simulink model "test_staticRelief"  (R2013a)
settings: Solver=ode15s  StartTime=0.0  StopTime=3  RelTol=1e-5
libraries: fl_lib x5, nesl_utility x3, simulink x2, usask_hyd_lib x1
settings Model: Creator=tkw954  LastModifiedBy=tkw954

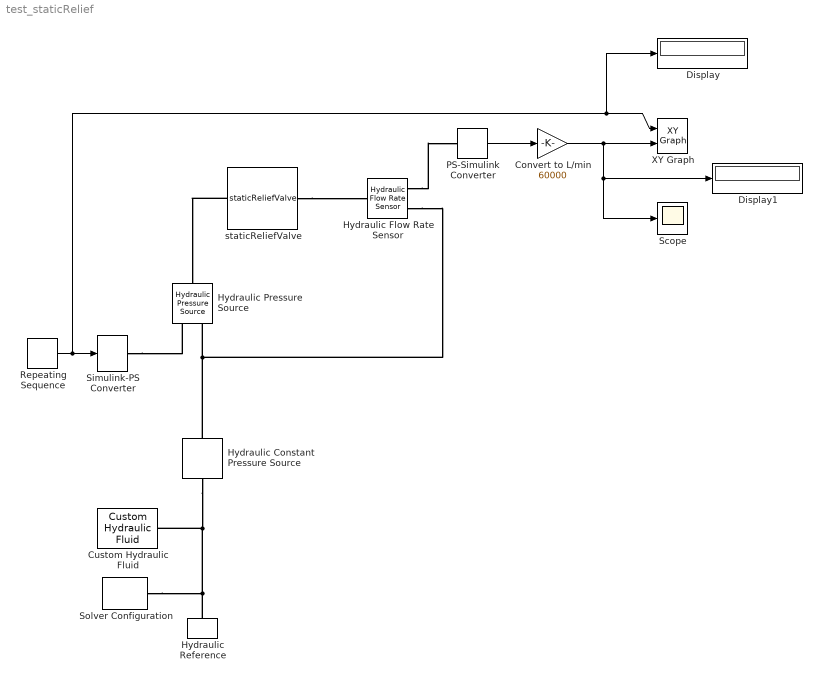
== system test_staticRelief ==
  Convert to L/min : Gain  Gain=60000
  Custom Hydraulic Fluid : fl_lib/Hydraulic/Hydraulic Utilities/Custom Hydraulic Fluid  density=850 kg/m^3  viscosity_kin=18e-6 m^2/s  bulk=0.8e9 Pa  alpha=0.005  LocalVarLogging=[]
  Display : Display
  Display1 : Display
  Hydraulic Constant Pressure Source : fl_lib/Hydraulic/Hydraulic Sources/Hydraulic Constant Pressure Source  commanded_pressure=10e6 Pa  pressure_Log=off  flow_rate_Log=off  power_Log=off  LocalVarNames=|pressure|flow_rate|power  LocalVarDescs=|Pressure differential|Flow rate|Power generated by the source  LocalVarLogging=[0 0 0]
  Hydraulic Flow Rate Sensor : fl_lib/Hydraulic/Hydraulic Sensors/Hydraulic Flow Rate Sensor  q_Log=off  p_Log=off  LocalVarNames=|q|p  LocalVarDescs=|q|p  LocalVarLogging=[0 0]
  Hydraulic Pressure Source : fl_lib/Hydraulic/Hydraulic Sources/Hydraulic Pressure Source  q_Log=off  p_Log=off  LocalVarNames=|q|p  LocalVarDescs=|q|p  LocalVarLogging=[0 0]
  Hydraulic Reference : fl_lib/Hydraulic/Hydraulic Elements/Hydraulic Reference  q_Log=off  LocalVarNames=|q  LocalVarDescs=|q  LocalVarLogging=0
  PS-Simulink Converter : nesl_utility/PS-Simulink Converter  PhysicalDomain=network_engine_domain  SubClassName=ps_output  LeftPortType=input  RightPortType=output  PseudoPeriodic=off  Frequencies=[]  Unit=1  AffineConversion=off
  Repeating Sequence : simulink/Sources/Repeating Sequence  rep_seq_t=[0 1 2 3]  rep_seq_y=[0 1 0 -1]*40e6
  Scope : Scope
  Simulink-PS Converter : nesl_utility/Simulink-PS Converter  PhysicalDomain=network_engine_domain  SubClassName=ps_input  LeftPortType=input  RightPortType=output  PseudoPeriodic=off  Frequencies=[]  NoiseDistribution=none  NoiseParameters=[]  Unit=1  AffineConversion=off  InputFiltering=off  SimscapeFilterOrder=1  InputFilterTimeConstant=0.001  UdotUserProvided=1
  Solver Configuration : nesl_utility/Solver Configuration  PhysicalDomain=network_engine_domain  SubClassName=solver  LeftPortType=input  RightPortType=generic  Accelerate=off  Tones=[]  Harmonics=[]  SimulateNoise=off  Profile=off  UseLocalSampling=off  EnableSwitchedLinearOptims=on  FrequencyDomain=off  UseCCode=off  UseNewInitialization=off  DoDC=off  ResidualTolerance=1e-09  UseLocalSolver=off  LocalSolverChoice=NE_BACKWARD_EULER_ADVANCER  LocalSolverSampleTime=0.001  DoFixedCost=off  MaxNonlinIter=3  MaxModeIter=2  LinearAlgebra=Sparse  DelaysMemoryBudget=1024
  XY Graph : simulink/Sinks/XY Graph  xmin=-10e6  xmax=30e6  ymin=-50  ymax=250  st=-1
  staticReliefValve : usask_hyd_lib/staticReliefValve  P_cr=10e6  P_or=1e6  A_max=20e-6  A_leak=1e-9  Cd=0.61
  wires:
  Repeating Sequence/1 -> Display/1, XY Graph/1, Simulink-PS Converter/1
  PS-Simulink Converter/1 -> Convert to L/min/1
  Convert to L/min/1 -> Display1/1, Scope/1, XY Graph/2
  connections:
  Hydraulic Reference/LConn1 -- Solver Configuration/RConn1 -- Hydraulic Constant Pressure Source/RConn1 -- Custom Hydraulic Fluid/RConn1
  Simulink-PS Converter/RConn1 -- Hydraulic Pressure Source/RConn1
  Hydraulic Flow Rate Sensor/RConn1 -- PS-Simulink Converter/LConn1
  Hydraulic Flow Rate Sensor/RConn2 -- Hydraulic Pressure Source/RConn2 -- Hydraulic Constant Pressure Source/LConn1
  staticReliefValve/RConn1 -- Hydraulic Flow Rate Sensor/LConn1
  staticReliefValve/LConn1 -- Hydraulic Pressure Source/LConn1
